simulink model "TST_InjVlv_BlkSht"  (R2016b)
settings: Solver=FixedStepDiscrete  StartTime=0.0  StopTime=simTime  FixedStep=sampleTime  RelTol=1e-3
values from neighbouring files (symbols this model uses):
  testCase = 1    [initTST_InjVlv_BlkSht_001.m]    (also in initTST_InjVlv_BlkSht_002.m = 2)
libraries: simulink x11, UnitTest_Lib x8
settings Model: Creator=zhengjinyan  LastModifiedBy=zhengjinyan
settings DebuggingCC: SignalRangeChecking=error

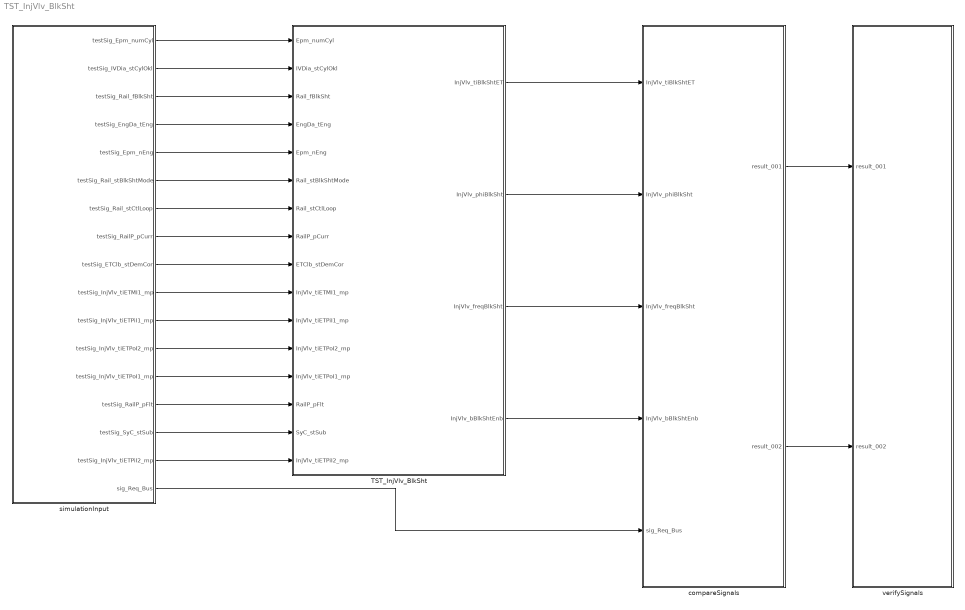
== system TST_InjVlv_BlkSht ==
  TST_InjVlv_BlkSht : Subsystem
  compareSignals : Subsystem
  simulationInput : Subsystem
  verifySignals : Subsystem
  wires:
  simulationInput/1(testSig_Epm_numCyl) -> TST_InjVlv_BlkSht/1(Epm_numCyl)
  simulationInput/2(testSig_IVDia_stCylOkl) -> TST_InjVlv_BlkSht/2(IVDia_stCylOkl)
  simulationInput/3(testSig_Rail_fBlkSht) -> TST_InjVlv_BlkSht/3(Rail_fBlkSht)
  simulationInput/4(testSig_EngDa_tEng) -> TST_InjVlv_BlkSht/4(EngDa_tEng)
  simulationInput/5(testSig_Epm_nEng) -> TST_InjVlv_BlkSht/5(Epm_nEng)
  simulationInput/6(testSig_Rail_stBlkShtMode) -> TST_InjVlv_BlkSht/6(Rail_stBlkShtMode)
  simulationInput/7(testSig_Rail_stCtlLoop) -> TST_InjVlv_BlkSht/7(Rail_stCtlLoop)
  simulationInput/8(testSig_RailP_pCurr) -> TST_InjVlv_BlkSht/8(RailP_pCurr)
  simulationInput/9(testSig_ETClb_stDemCor) -> TST_InjVlv_BlkSht/9(ETClb_stDemCor)
  simulationInput/10(testSig_InjVlv_tiETMI1_mp) -> TST_InjVlv_BlkSht/10(InjVlv_tiETMI1_mp)
  simulationInput/11(testSig_InjVlv_tiETPiI1_mp) -> TST_InjVlv_BlkSht/11(InjVlv_tiETPiI1_mp)
  simulationInput/12(testSig_InjVlv_tiETPoI2_mp) -> TST_InjVlv_BlkSht/12(InjVlv_tiETPoI2_mp)
  simulationInput/13(testSig_InjVlv_tiETPoI1_mp) -> TST_InjVlv_BlkSht/13(InjVlv_tiETPoI1_mp)
  simulationInput/14(testSig_RailP_pFlt) -> TST_InjVlv_BlkSht/14(RailP_pFlt)
  simulationInput/15(testSig_SyC_stSub) -> TST_InjVlv_BlkSht/15(SyC_stSub)
  simulationInput/16(testSig_InjVlv_tiETPiI2_mp) -> TST_InjVlv_BlkSht/16(InjVlv_tiETPiI2_mp)
  TST_InjVlv_BlkSht/1(InjVlv_tiBlkShtET) -> compareSignals/1(InjVlv_tiBlkShtET)
  TST_InjVlv_BlkSht/2(InjVlv_phiBlkSht) -> compareSignals/2(InjVlv_phiBlkSht)
  TST_InjVlv_BlkSht/3(InjVlv_freqBlkSht) -> compareSignals/3(InjVlv_freqBlkSht)
  TST_InjVlv_BlkSht/4(InjVlv_bBlkShtEnb) -> compareSignals/4(InjVlv_bBlkShtEnb)
  simulationInput/17(sig_Req_Bus) -> compareSignals/5(sig_Req_Bus)
  compareSignals/1(result_001) -> verifySignals/1(result_001)
  compareSignals/2(result_002) -> verifySignals/2(result_002)

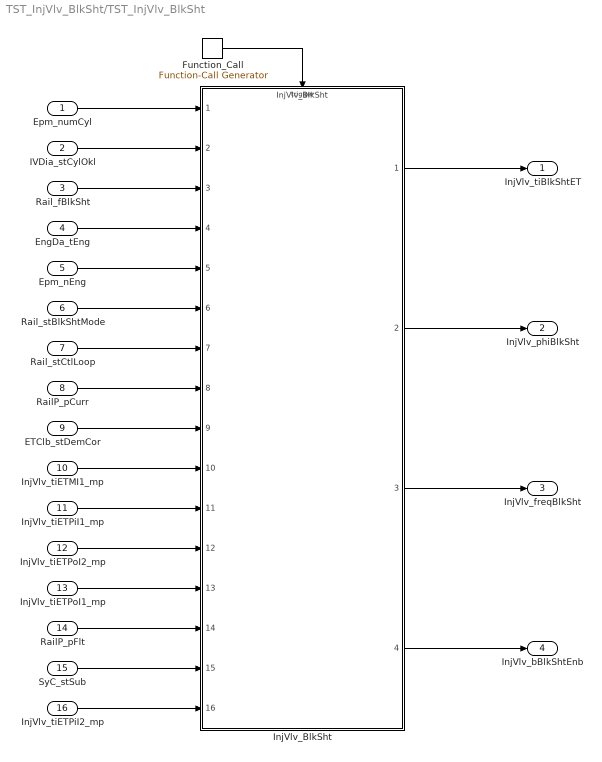
== system TST_InjVlv_BlkSht/TST_InjVlv_BlkSht ==
  Epm_numCyl : Inport
  IVDia_stCylOkl : Inport  Port=2
  Rail_fBlkSht : Inport  Port=3
  EngDa_tEng : Inport  Port=4
  Epm_nEng : Inport  Port=5
  Rail_stBlkShtMode : Inport  Port=6
  Rail_stCtlLoop : Inport  Port=7
  RailP_pCurr : Inport  Port=8
  ETClb_stDemCor : Inport  Port=9
  InjVlv_tiETMI1_mp : Inport  Port=10
  InjVlv_tiETPiI1_mp : Inport  Port=11
  InjVlv_tiETPoI2_mp : Inport  Port=12
  InjVlv_tiETPoI1_mp : Inport  Port=13
  RailP_pFlt : Inport  Port=14
  SyC_stSub : Inport  Port=15
  InjVlv_tiETPiI2_mp : Inport  Port=16
  Function_Call : simulink/Ports & Subsystems/Function-Call Generator  sample_time=sampleTime  numberOfIterations=1
  InjVlv_BlkSht : ModelReference  ModelNameDialog=InjVlv_BlkSht  SimulationMode=Normal  ModelReferenceVersion=1.63  TriggerPortName=function  TriggerPortTriggerType=function-call  TriggerPortStatesWhenEnabling=held
  InjVlv_tiBlkShtET : Outport
  InjVlv_phiBlkSht : Outport  Port=2
  InjVlv_freqBlkSht : Outport  Port=3
  InjVlv_bBlkShtEnb : Outport  Port=4
  wires:
  Function_Call/1 -> InjVlv_BlkSht/Trigger
  Epm_numCyl/1 -> InjVlv_BlkSht/1
  IVDia_stCylOkl/1 -> InjVlv_BlkSht/2
  Rail_fBlkSht/1 -> InjVlv_BlkSht/3
  EngDa_tEng/1 -> InjVlv_BlkSht/4
  Epm_nEng/1 -> InjVlv_BlkSht/5
  Rail_stBlkShtMode/1 -> InjVlv_BlkSht/6
  Rail_stCtlLoop/1 -> InjVlv_BlkSht/7
  RailP_pCurr/1 -> InjVlv_BlkSht/8
  ETClb_stDemCor/1 -> InjVlv_BlkSht/9
  InjVlv_tiETMI1_mp/1 -> InjVlv_BlkSht/10
  InjVlv_tiETPiI1_mp/1 -> InjVlv_BlkSht/11
  InjVlv_tiETPoI2_mp/1 -> InjVlv_BlkSht/12
  InjVlv_tiETPoI1_mp/1 -> InjVlv_BlkSht/13
  RailP_pFlt/1 -> InjVlv_BlkSht/14
  SyC_stSub/1 -> InjVlv_BlkSht/15
  InjVlv_tiETPiI2_mp/1 -> InjVlv_BlkSht/16
  InjVlv_BlkSht/1 -> InjVlv_tiBlkShtET/1
  InjVlv_BlkSht/2 -> InjVlv_phiBlkSht/1
  InjVlv_BlkSht/3 -> InjVlv_freqBlkSht/1
  InjVlv_BlkSht/4 -> InjVlv_bBlkShtEnb/1

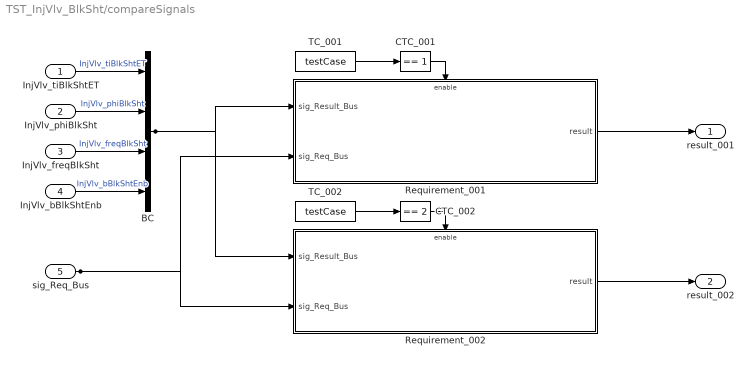
== system TST_InjVlv_BlkSht/compareSignals ==
  InjVlv_tiBlkShtET : Inport
  InjVlv_phiBlkSht : Inport  Port=2
  InjVlv_freqBlkSht : Inport  Port=3
  InjVlv_bBlkShtEnb : Inport  Port=4
  sig_Req_Bus : Inport  Port=5
  BC : BusCreator  Inputs=4
  CTC_001 : simulink/Logic and Bit Operations/Compare To Constant  relop===  const=1  OutDataTypeStr=boolean
  CTC_002 : simulink/Logic and Bit Operations/Compare To Constant  relop===  const=2  OutDataTypeStr=boolean
  Requirement_001 : Subsystem
  Requirement_002 : Subsystem
  TC_001 : Constant  Value=testCase
  TC_002 : Constant  Value=testCase
  result_001 : Outport
  result_002 : Outport  Port=2
  wires:
  InjVlv_tiBlkShtET/1 -> BC/1  "InjVlv_tiBlkShtET"
  InjVlv_phiBlkSht/1 -> BC/2  "InjVlv_phiBlkSht"
  InjVlv_freqBlkSht/1 -> BC/3  "InjVlv_freqBlkSht"
  InjVlv_bBlkShtEnb/1 -> BC/4  "InjVlv_bBlkShtEnb"
  TC_001/1 -> CTC_001/1
  CTC_001/1 -> Requirement_001/Enable
  sig_Req_Bus/1 -> Requirement_001/2(sig_Req_Bus), Requirement_002/2(sig_Req_Bus)
  BC/1 -> Requirement_001/1(sig_Result_Bus), Requirement_002/1(sig_Result_Bus)
  Requirement_001/1(result) -> result_001/1
  TC_002/1 -> CTC_002/1
  CTC_002/1 -> Requirement_002/Enable
  Requirement_002/1(result) -> result_002/1

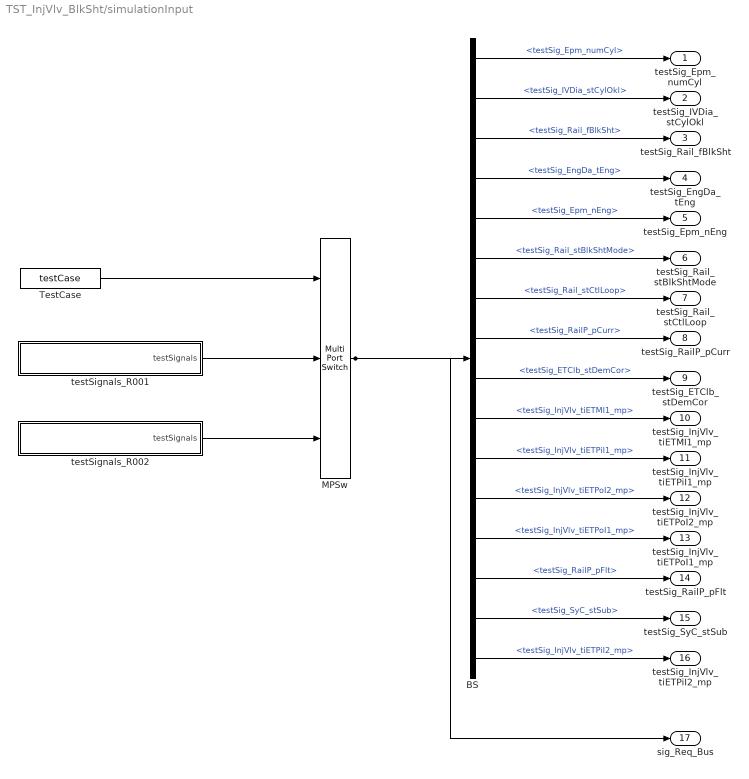
== system TST_InjVlv_BlkSht/simulationInput ==
  BS : BusSelector  OutputSignals=testSig_Epm_numCyl,testSig_IVDia_stCylOkl,testSig_Rail_fBlkSht,testSig_EngDa_tEng,testSig_Epm_nEng,testSig_Rail_stBlkShtMode,testSig_Rail_stCtlLoop,testSig_RailP_pCurr,testSig_ETClb_stDemCor,testSig_InjVlv_tiETMI1_mp,testSig_InjVlv_tiETPiI1_mp,testSig_InjVlv_tiETPoI2_mp,testSig_InjVlv_tiETPoI1_mp,testSig_RailP_pFlt,testSig_SyC_stSub,testSig_InjVlv_tiETPiI2_mp
  MPSw : MultiPortSwitch  Inputs=2  SaturateOnIntegerOverflow=on  InputSameDT=on
  TestCase : Constant  Value=testCase
  testSignals_R001 : Subsystem
  testSignals_R002 : Subsystem
  testSig_Epm_numCyl : Outport
  testSig_IVDia_stCylOkl : Outport  Port=2
  testSig_Rail_fBlkSht : Outport  Port=3
  testSig_EngDa_tEng : Outport  Port=4
  testSig_Epm_nEng : Outport  Port=5
  testSig_Rail_stBlkShtMode : Outport  Port=6
  testSig_Rail_stCtlLoop : Outport  Port=7
  testSig_RailP_pCurr : Outport  Port=8
  testSig_ETClb_stDemCor : Outport  Port=9
  testSig_InjVlv_tiETMI1_mp : Outport  Port=10
  testSig_InjVlv_tiETPiI1_mp : Outport  Port=11
  testSig_InjVlv_tiETPoI2_mp : Outport  Port=12
  testSig_InjVlv_tiETPoI1_mp : Outport  Port=13
  testSig_RailP_pFlt : Outport  Port=14
  testSig_SyC_stSub : Outport  Port=15
  testSig_InjVlv_tiETPiI2_mp : Outport  Port=16
  sig_Req_Bus : Outport  Port=17
  wires:
  BS/1 -> testSig_Epm_numCyl/1  "<testSig_Epm_numCyl>"
  BS/2 -> testSig_IVDia_stCylOkl/1  "<testSig_IVDia_stCylOkl>"
  BS/3 -> testSig_Rail_fBlkSht/1  "<testSig_Rail_fBlkSht>"
  BS/4 -> testSig_EngDa_tEng/1  "<testSig_EngDa_tEng>"
  BS/5 -> testSig_Epm_nEng/1  "<testSig_Epm_nEng>"
  BS/6 -> testSig_Rail_stBlkShtMode/1  "<testSig_Rail_stBlkShtMode>"
  BS/7 -> testSig_Rail_stCtlLoop/1  "<testSig_Rail_stCtlLoop>"
  BS/8 -> testSig_RailP_pCurr/1  "<testSig_RailP_pCurr>"
  BS/9 -> testSig_ETClb_stDemCor/1  "<testSig_ETClb_stDemCor>"
  BS/10 -> testSig_InjVlv_tiETMI1_mp/1  "<testSig_InjVlv_tiETMI1_mp>"
  BS/11 -> testSig_InjVlv_tiETPiI1_mp/1  "<testSig_InjVlv_tiETPiI1_mp>"
  BS/12 -> testSig_InjVlv_tiETPoI2_mp/1  "<testSig_InjVlv_tiETPoI2_mp>"
  BS/13 -> testSig_InjVlv_tiETPoI1_mp/1  "<testSig_InjVlv_tiETPoI1_mp>"
  BS/14 -> testSig_RailP_pFlt/1  "<testSig_RailP_pFlt>"
  BS/15 -> testSig_SyC_stSub/1  "<testSig_SyC_stSub>"
  BS/16 -> testSig_InjVlv_tiETPiI2_mp/1  "<testSig_InjVlv_tiETPiI2_mp>"
  MPSw/1 -> BS/1, sig_Req_Bus/1
  TestCase/1 -> MPSw/1
  testSignals_R001/1(testSignals) -> MPSw/2
  testSignals_R002/1(testSignals) -> MPSw/3

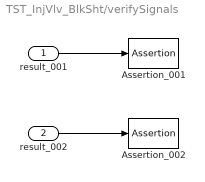
== system TST_InjVlv_BlkSht/verifySignals ==
  result_001 : Inport
  result_002 : Inport  Port=2
  Assertion_001 : Assertion  Enabled=off
  Assertion_002 : Assertion  Enabled=off
  wires:
  result_001/1 -> Assertion_001/1
  result_002/1 -> Assertion_002/1

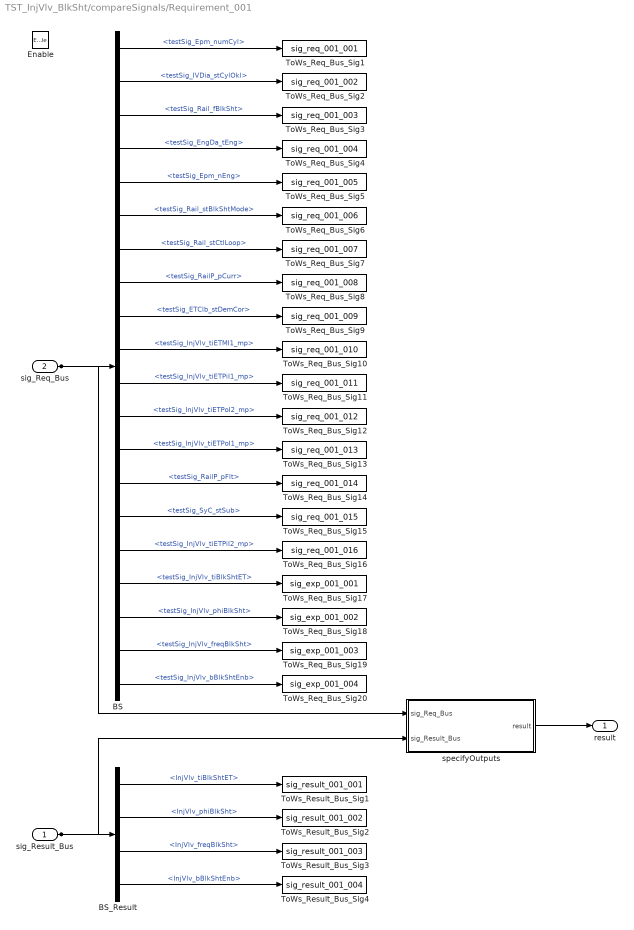
== system TST_InjVlv_BlkSht/compareSignals/Requirement_001 ==
  sig_Result_Bus : Inport
  sig_Req_Bus : Inport  Port=2
  Enable : EnablePort
  BS : BusSelector  OutputSignals=testSig_Epm_numCyl,testSig_IVDia_stCylOkl,testSig_Rail_fBlkSht,testSig_EngDa_tEng,testSig_Epm_nEng,testSig_Rail_stBlkShtMode,testSig_Rail_stCtlLoop,testSig_RailP_pCurr,testSig_ETClb_stDemCor,testSig_InjVlv_tiETMI1_mp,testSig_InjVlv_tiETPiI1_mp,testSig_InjVlv_tiETPoI2_mp,testSig_InjVlv_tiETPoI1_mp,testSig_RailP_pFlt,testSig_SyC_stSub,testSig_InjVlv_tiETPiI2_mp,testSig_InjVlv_tiBlkShtET,testSig_InjVlv_phiBlkSht,testSig_InjVlv_freqBlkSht,testSig_InjVlv_bBlkShtEnb
  BS_Result : BusSelector  OutputSignals=InjVlv_tiBlkShtET,InjVlv_phiBlkSht,InjVlv_freqBlkSht,InjVlv_bBlkShtEnb
  ToWs_Req_Bus_Sig1 : ToWorkspace  VariableName=sig_req_001_001  SaveFormat=Structure With Time
  ToWs_Req_Bus_Sig10 : ToWorkspace  VariableName=sig_req_001_010  SaveFormat=Structure With Time
  ToWs_Req_Bus_Sig11 : ToWorkspace  VariableName=sig_req_001_011  SaveFormat=Structure With Time
  ToWs_Req_Bus_Sig12 : ToWorkspace  VariableName=sig_req_001_012  SaveFormat=Structure With Time
  ToWs_Req_Bus_Sig13 : ToWorkspace  VariableName=sig_req_001_013  SaveFormat=Structure With Time
  ToWs_Req_Bus_Sig14 : ToWorkspace  VariableName=sig_req_001_014  SaveFormat=Structure With Time
  ToWs_Req_Bus_Sig15 : ToWorkspace  VariableName=sig_req_001_015  SaveFormat=Structure With Time
  ToWs_Req_Bus_Sig16 : ToWorkspace  VariableName=sig_req_001_016  SaveFormat=Structure With Time
  ToWs_Req_Bus_Sig17 : ToWorkspace  VariableName=sig_exp_001_001  SaveFormat=Structure With Time
  ToWs_Req_Bus_Sig18 : ToWorkspace  VariableName=sig_exp_001_002  SaveFormat=Structure With Time
  ToWs_Req_Bus_Sig19 : ToWorkspace  VariableName=sig_exp_001_003  SaveFormat=Structure With Time
  ToWs_Req_Bus_Sig2 : ToWorkspace  VariableName=sig_req_001_002  SaveFormat=Structure With Time
  ToWs_Req_Bus_Sig20 : ToWorkspace  VariableName=sig_exp_001_004  SaveFormat=Structure With Time
  ToWs_Req_Bus_Sig3 : ToWorkspace  VariableName=sig_req_001_003  SaveFormat=Structure With Time
  ToWs_Req_Bus_Sig4 : ToWorkspace  VariableName=sig_req_001_004  SaveFormat=Structure With Time
  ToWs_Req_Bus_Sig5 : ToWorkspace  VariableName=sig_req_001_005  SaveFormat=Structure With Time
  ToWs_Req_Bus_Sig6 : ToWorkspace  VariableName=sig_req_001_006  SaveFormat=Structure With Time
  ToWs_Req_Bus_Sig7 : ToWorkspace  VariableName=sig_req_001_007  SaveFormat=Structure With Time
  ToWs_Req_Bus_Sig8 : ToWorkspace  VariableName=sig_req_001_008  SaveFormat=Structure With Time
  ToWs_Req_Bus_Sig9 : ToWorkspace  VariableName=sig_req_001_009  SaveFormat=Structure With Time
  ToWs_Result_Bus_Sig1 : ToWorkspace  VariableName=sig_result_001_001  SaveFormat=Structure With Time
  ToWs_Result_Bus_Sig2 : ToWorkspace  VariableName=sig_result_001_002  SaveFormat=Structure With Time
  ToWs_Result_Bus_Sig3 : ToWorkspace  VariableName=sig_result_001_003  SaveFormat=Structure With Time
  ToWs_Result_Bus_Sig4 : ToWorkspace  VariableName=sig_result_001_004  SaveFormat=Structure With Time
  specifyOutputs : Subsystem
  result : Outport
  wires:
  sig_Req_Bus/1 -> BS/1, specifyOutputs/1(sig_Req_Bus)
  BS/1 -> ToWs_Req_Bus_Sig1/1  "<testSig_Epm_numCyl>"
  BS/2 -> ToWs_Req_Bus_Sig2/1  "<testSig_IVDia_stCylOkl>"
  BS/3 -> ToWs_Req_Bus_Sig3/1  "<testSig_Rail_fBlkSht>"
  BS/4 -> ToWs_Req_Bus_Sig4/1  "<testSig_EngDa_tEng>"
  BS/5 -> ToWs_Req_Bus_Sig5/1  "<testSig_Epm_nEng>"
  BS/6 -> ToWs_Req_Bus_Sig6/1  "<testSig_Rail_stBlkShtMode>"
  BS/7 -> ToWs_Req_Bus_Sig7/1  "<testSig_Rail_stCtlLoop>"
  BS/8 -> ToWs_Req_Bus_Sig8/1  "<testSig_RailP_pCurr>"
  BS/9 -> ToWs_Req_Bus_Sig9/1  "<testSig_ETClb_stDemCor>"
  BS/10 -> ToWs_Req_Bus_Sig10/1  "<testSig_InjVlv_tiETMI1_mp>"
  BS/11 -> ToWs_Req_Bus_Sig11/1  "<testSig_InjVlv_tiETPiI1_mp>"
  BS/12 -> ToWs_Req_Bus_Sig12/1  "<testSig_InjVlv_tiETPoI2_mp>"
  BS/13 -> ToWs_Req_Bus_Sig13/1  "<testSig_InjVlv_tiETPoI1_mp>"
  BS/14 -> ToWs_Req_Bus_Sig14/1  "<testSig_RailP_pFlt>"
  BS/15 -> ToWs_Req_Bus_Sig15/1  "<testSig_SyC_stSub>"
  BS/16 -> ToWs_Req_Bus_Sig16/1  "<testSig_InjVlv_tiETPiI2_mp>"
  BS/17 -> ToWs_Req_Bus_Sig17/1  "<testSig_InjVlv_tiBlkShtET>"
  BS/18 -> ToWs_Req_Bus_Sig18/1  "<testSig_InjVlv_phiBlkSht>"
  BS/19 -> ToWs_Req_Bus_Sig19/1  "<testSig_InjVlv_freqBlkSht>"
  BS/20 -> ToWs_Req_Bus_Sig20/1  "<testSig_InjVlv_bBlkShtEnb>"
  sig_Result_Bus/1 -> BS_Result/1, specifyOutputs/2(sig_Result_Bus)
  BS_Result/1 -> ToWs_Result_Bus_Sig1/1  "<InjVlv_tiBlkShtET>"
  BS_Result/2 -> ToWs_Result_Bus_Sig2/1  "<InjVlv_phiBlkSht>"
  BS_Result/3 -> ToWs_Result_Bus_Sig3/1  "<InjVlv_freqBlkSht>"
  BS_Result/4 -> ToWs_Result_Bus_Sig4/1  "<InjVlv_bBlkShtEnb>"
  specifyOutputs/1(result) -> result/1

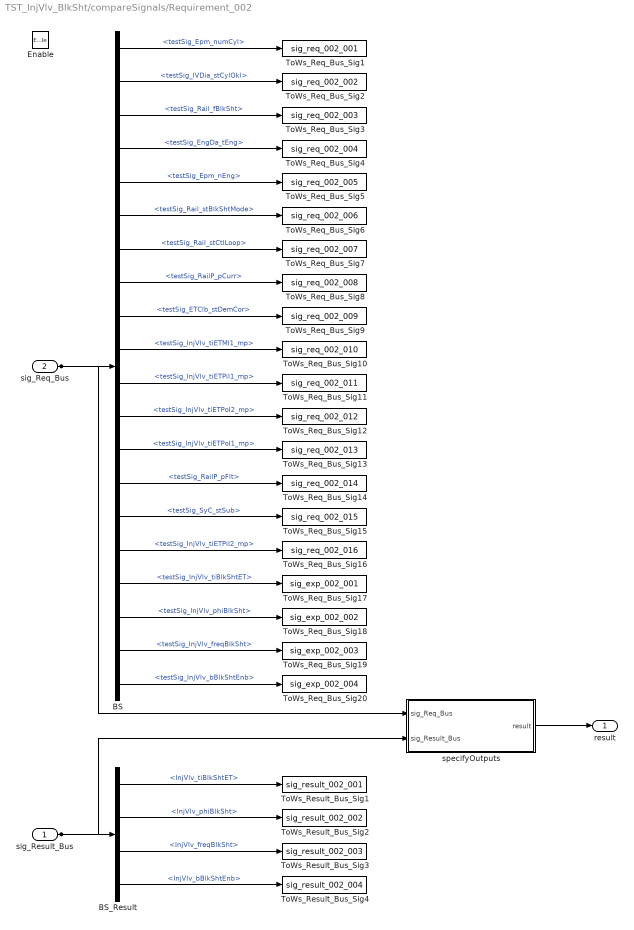
== system TST_InjVlv_BlkSht/compareSignals/Requirement_002 ==
  sig_Result_Bus : Inport
  sig_Req_Bus : Inport  Port=2
  Enable : EnablePort
  BS : BusSelector  OutputSignals=testSig_Epm_numCyl,testSig_IVDia_stCylOkl,testSig_Rail_fBlkSht,testSig_EngDa_tEng,testSig_Epm_nEng,testSig_Rail_stBlkShtMode,testSig_Rail_stCtlLoop,testSig_RailP_pCurr,testSig_ETClb_stDemCor,testSig_InjVlv_tiETMI1_mp,testSig_InjVlv_tiETPiI1_mp,testSig_InjVlv_tiETPoI2_mp,testSig_InjVlv_tiETPoI1_mp,testSig_RailP_pFlt,testSig_SyC_stSub,testSig_InjVlv_tiETPiI2_mp,testSig_InjVlv_tiBlkShtET,testSig_InjVlv_phiBlkSht,testSig_InjVlv_freqBlkSht,testSig_InjVlv_bBlkShtEnb
  BS_Result : BusSelector  OutputSignals=InjVlv_tiBlkShtET,InjVlv_phiBlkSht,InjVlv_freqBlkSht,InjVlv_bBlkShtEnb
  ToWs_Req_Bus_Sig1 : ToWorkspace  VariableName=sig_req_002_001  SaveFormat=Structure With Time
  ToWs_Req_Bus_Sig10 : ToWorkspace  VariableName=sig_req_002_010  SaveFormat=Structure With Time
  ToWs_Req_Bus_Sig11 : ToWorkspace  VariableName=sig_req_002_011  SaveFormat=Structure With Time
  ToWs_Req_Bus_Sig12 : ToWorkspace  VariableName=sig_req_002_012  SaveFormat=Structure With Time
  ToWs_Req_Bus_Sig13 : ToWorkspace  VariableName=sig_req_002_013  SaveFormat=Structure With Time
  ToWs_Req_Bus_Sig14 : ToWorkspace  VariableName=sig_req_002_014  SaveFormat=Structure With Time
  ToWs_Req_Bus_Sig15 : ToWorkspace  VariableName=sig_req_002_015  SaveFormat=Structure With Time
  ToWs_Req_Bus_Sig16 : ToWorkspace  VariableName=sig_req_002_016  SaveFormat=Structure With Time
  ToWs_Req_Bus_Sig17 : ToWorkspace  VariableName=sig_exp_002_001  SaveFormat=Structure With Time
  ToWs_Req_Bus_Sig18 : ToWorkspace  VariableName=sig_exp_002_002  SaveFormat=Structure With Time
  ToWs_Req_Bus_Sig19 : ToWorkspace  VariableName=sig_exp_002_003  SaveFormat=Structure With Time
  ToWs_Req_Bus_Sig2 : ToWorkspace  VariableName=sig_req_002_002  SaveFormat=Structure With Time
  ToWs_Req_Bus_Sig20 : ToWorkspace  VariableName=sig_exp_002_004  SaveFormat=Structure With Time
  ToWs_Req_Bus_Sig3 : ToWorkspace  VariableName=sig_req_002_003  SaveFormat=Structure With Time
  ToWs_Req_Bus_Sig4 : ToWorkspace  VariableName=sig_req_002_004  SaveFormat=Structure With Time
  ToWs_Req_Bus_Sig5 : ToWorkspace  VariableName=sig_req_002_005  SaveFormat=Structure With Time
  ToWs_Req_Bus_Sig6 : ToWorkspace  VariableName=sig_req_002_006  SaveFormat=Structure With Time
  ToWs_Req_Bus_Sig7 : ToWorkspace  VariableName=sig_req_002_007  SaveFormat=Structure With Time
  ToWs_Req_Bus_Sig8 : ToWorkspace  VariableName=sig_req_002_008  SaveFormat=Structure With Time
  ToWs_Req_Bus_Sig9 : ToWorkspace  VariableName=sig_req_002_009  SaveFormat=Structure With Time
  ToWs_Result_Bus_Sig1 : ToWorkspace  VariableName=sig_result_002_001  SaveFormat=Structure With Time
  ToWs_Result_Bus_Sig2 : ToWorkspace  VariableName=sig_result_002_002  SaveFormat=Structure With Time
  ToWs_Result_Bus_Sig3 : ToWorkspace  VariableName=sig_result_002_003  SaveFormat=Structure With Time
  ToWs_Result_Bus_Sig4 : ToWorkspace  VariableName=sig_result_002_004  SaveFormat=Structure With Time
  specifyOutputs : Subsystem
  result : Outport
  wires:
  sig_Req_Bus/1 -> BS/1, specifyOutputs/1(sig_Req_Bus)
  BS/1 -> ToWs_Req_Bus_Sig1/1  "<testSig_Epm_numCyl>"
  BS/2 -> ToWs_Req_Bus_Sig2/1  "<testSig_IVDia_stCylOkl>"
  BS/3 -> ToWs_Req_Bus_Sig3/1  "<testSig_Rail_fBlkSht>"
  BS/4 -> ToWs_Req_Bus_Sig4/1  "<testSig_EngDa_tEng>"
  BS/5 -> ToWs_Req_Bus_Sig5/1  "<testSig_Epm_nEng>"
  BS/6 -> ToWs_Req_Bus_Sig6/1  "<testSig_Rail_stBlkShtMode>"
  BS/7 -> ToWs_Req_Bus_Sig7/1  "<testSig_Rail_stCtlLoop>"
  BS/8 -> ToWs_Req_Bus_Sig8/1  "<testSig_RailP_pCurr>"
  BS/9 -> ToWs_Req_Bus_Sig9/1  "<testSig_ETClb_stDemCor>"
  BS/10 -> ToWs_Req_Bus_Sig10/1  "<testSig_InjVlv_tiETMI1_mp>"
  BS/11 -> ToWs_Req_Bus_Sig11/1  "<testSig_InjVlv_tiETPiI1_mp>"
  BS/12 -> ToWs_Req_Bus_Sig12/1  "<testSig_InjVlv_tiETPoI2_mp>"
  BS/13 -> ToWs_Req_Bus_Sig13/1  "<testSig_InjVlv_tiETPoI1_mp>"
  BS/14 -> ToWs_Req_Bus_Sig14/1  "<testSig_RailP_pFlt>"
  BS/15 -> ToWs_Req_Bus_Sig15/1  "<testSig_SyC_stSub>"
  BS/16 -> ToWs_Req_Bus_Sig16/1  "<testSig_InjVlv_tiETPiI2_mp>"
  BS/17 -> ToWs_Req_Bus_Sig17/1  "<testSig_InjVlv_tiBlkShtET>"
  BS/18 -> ToWs_Req_Bus_Sig18/1  "<testSig_InjVlv_phiBlkSht>"
  BS/19 -> ToWs_Req_Bus_Sig19/1  "<testSig_InjVlv_freqBlkSht>"
  BS/20 -> ToWs_Req_Bus_Sig20/1  "<testSig_InjVlv_bBlkShtEnb>"
  sig_Result_Bus/1 -> BS_Result/1, specifyOutputs/2(sig_Result_Bus)
  BS_Result/1 -> ToWs_Result_Bus_Sig1/1  "<InjVlv_tiBlkShtET>"
  BS_Result/2 -> ToWs_Result_Bus_Sig2/1  "<InjVlv_phiBlkSht>"
  BS_Result/3 -> ToWs_Result_Bus_Sig3/1  "<InjVlv_freqBlkSht>"
  BS_Result/4 -> ToWs_Result_Bus_Sig4/1  "<InjVlv_bBlkShtEnb>"
  specifyOutputs/1(result) -> result/1

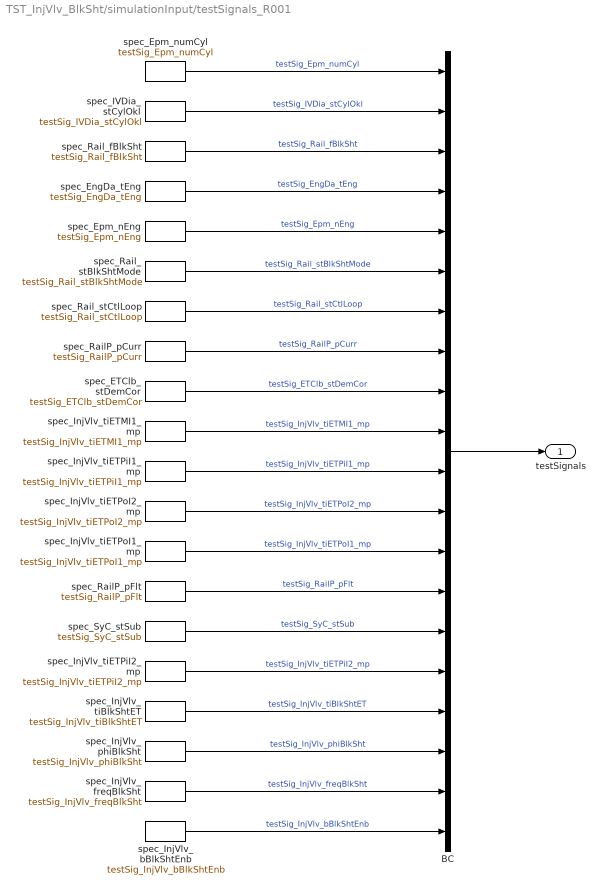
== system TST_InjVlv_BlkSht/simulationInput/testSignals_R001 ==
  BC : BusCreator  Inputs=20
  spec_ETClb_stDemCor : FromWorkspace  VariableName=testSig_ETClb_stDemCor  Interpolate=off  OutputAfterFinalValue=Holding final value
  spec_EngDa_tEng : FromWorkspace  VariableName=testSig_EngDa_tEng  Interpolate=off  OutputAfterFinalValue=Holding final value
  spec_Epm_nEng : FromWorkspace  VariableName=testSig_Epm_nEng  Interpolate=off  OutputAfterFinalValue=Holding final value
  spec_Epm_numCyl : FromWorkspace  VariableName=testSig_Epm_numCyl  Interpolate=off  OutputAfterFinalValue=Holding final value
  spec_IVDia_stCylOkl : FromWorkspace  VariableName=testSig_IVDia_stCylOkl  Interpolate=off  OutputAfterFinalValue=Holding final value
  spec_InjVlv_bBlkShtEnb : FromWorkspace  VariableName=testSig_InjVlv_bBlkShtEnb  Interpolate=off  OutputAfterFinalValue=Holding final value
  spec_InjVlv_freqBlkSht : FromWorkspace  VariableName=testSig_InjVlv_freqBlkSht  Interpolate=off  OutputAfterFinalValue=Holding final value
  spec_InjVlv_phiBlkSht : FromWorkspace  VariableName=testSig_InjVlv_phiBlkSht  Interpolate=off  OutputAfterFinalValue=Holding final value
  spec_InjVlv_tiBlkShtET : FromWorkspace  VariableName=testSig_InjVlv_tiBlkShtET  Interpolate=off  OutputAfterFinalValue=Holding final value
  spec_InjVlv_tiETMI1_mp : FromWorkspace  VariableName=testSig_InjVlv_tiETMI1_mp  Interpolate=off  OutputAfterFinalValue=Holding final value
  spec_InjVlv_tiETPiI1_mp : FromWorkspace  VariableName=testSig_InjVlv_tiETPiI1_mp  Interpolate=off  OutputAfterFinalValue=Holding final value
  spec_InjVlv_tiETPiI2_mp : FromWorkspace  VariableName=testSig_InjVlv_tiETPiI2_mp  Interpolate=off  OutputAfterFinalValue=Holding final value
  spec_InjVlv_tiETPoI1_mp : FromWorkspace  VariableName=testSig_InjVlv_tiETPoI1_mp  Interpolate=off  OutputAfterFinalValue=Holding final value
  spec_InjVlv_tiETPoI2_mp : FromWorkspace  VariableName=testSig_InjVlv_tiETPoI2_mp  Interpolate=off  OutputAfterFinalValue=Holding final value
  spec_RailP_pCurr : FromWorkspace  VariableName=testSig_RailP_pCurr  Interpolate=off  OutputAfterFinalValue=Holding final value
  spec_RailP_pFlt : FromWorkspace  VariableName=testSig_RailP_pFlt  Interpolate=off  OutputAfterFinalValue=Holding final value
  spec_Rail_fBlkSht : FromWorkspace  VariableName=testSig_Rail_fBlkSht  Interpolate=off  OutputAfterFinalValue=Holding final value
  spec_Rail_stBlkShtMode : FromWorkspace  VariableName=testSig_Rail_stBlkShtMode  Interpolate=off  OutputAfterFinalValue=Holding final value
  spec_Rail_stCtlLoop : FromWorkspace  VariableName=testSig_Rail_stCtlLoop  Interpolate=off  OutputAfterFinalValue=Holding final value
  spec_SyC_stSub : FromWorkspace  VariableName=testSig_SyC_stSub  Interpolate=off  OutputAfterFinalValue=Holding final value
  testSignals : Outport
  wires:
  BC/1 -> testSignals/1
  spec_Epm_numCyl/1 -> BC/1  "testSig_Epm_numCyl"
  spec_IVDia_stCylOkl/1 -> BC/2  "testSig_IVDia_stCylOkl"
  spec_Rail_fBlkSht/1 -> BC/3  "testSig_Rail_fBlkSht"
  spec_EngDa_tEng/1 -> BC/4  "testSig_EngDa_tEng"
  spec_Epm_nEng/1 -> BC/5  "testSig_Epm_nEng"
  spec_Rail_stBlkShtMode/1 -> BC/6  "testSig_Rail_stBlkShtMode"
  spec_Rail_stCtlLoop/1 -> BC/7  "testSig_Rail_stCtlLoop"
  spec_RailP_pCurr/1 -> BC/8  "testSig_RailP_pCurr"
  spec_ETClb_stDemCor/1 -> BC/9  "testSig_ETClb_stDemCor"
  spec_InjVlv_tiETMI1_mp/1 -> BC/10  "testSig_InjVlv_tiETMI1_mp"
  spec_InjVlv_tiETPiI1_mp/1 -> BC/11  "testSig_InjVlv_tiETPiI1_mp"
  spec_InjVlv_tiETPoI2_mp/1 -> BC/12  "testSig_InjVlv_tiETPoI2_mp"
  spec_InjVlv_tiETPoI1_mp/1 -> BC/13  "testSig_InjVlv_tiETPoI1_mp"
  spec_RailP_pFlt/1 -> BC/14  "testSig_RailP_pFlt"
  spec_SyC_stSub/1 -> BC/15  "testSig_SyC_stSub"
  spec_InjVlv_tiETPiI2_mp/1 -> BC/16  "testSig_InjVlv_tiETPiI2_mp"
  spec_InjVlv_tiBlkShtET/1 -> BC/17  "testSig_InjVlv_tiBlkShtET"
  spec_InjVlv_phiBlkSht/1 -> BC/18  "testSig_InjVlv_phiBlkSht"
  spec_InjVlv_freqBlkSht/1 -> BC/19  "testSig_InjVlv_freqBlkSht"
  spec_InjVlv_bBlkShtEnb/1 -> BC/20  "testSig_InjVlv_bBlkShtEnb"

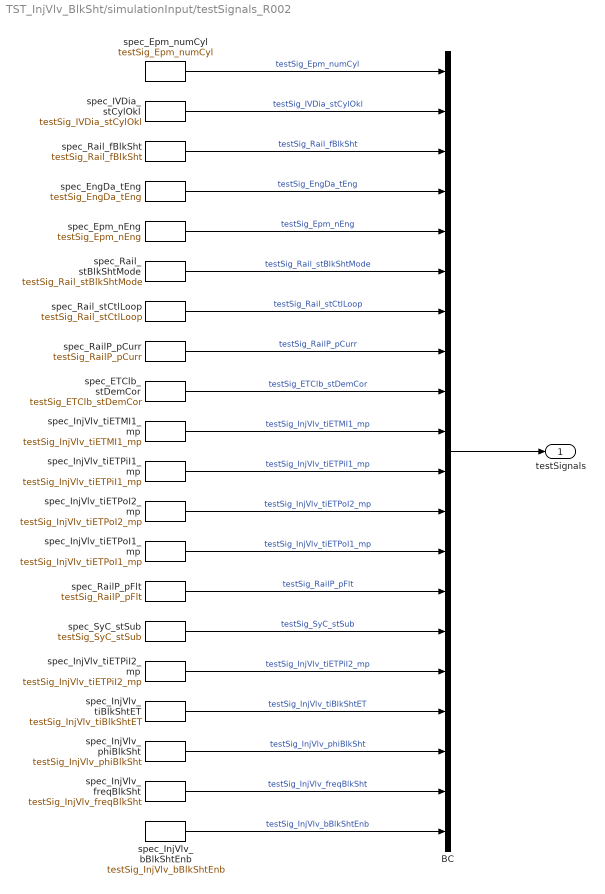
== system TST_InjVlv_BlkSht/simulationInput/testSignals_R002 ==
  BC : BusCreator  Inputs=20
  spec_ETClb_stDemCor : FromWorkspace  VariableName=testSig_ETClb_stDemCor  Interpolate=off  OutputAfterFinalValue=Holding final value
  spec_EngDa_tEng : FromWorkspace  VariableName=testSig_EngDa_tEng  Interpolate=off  OutputAfterFinalValue=Holding final value
  spec_Epm_nEng : FromWorkspace  VariableName=testSig_Epm_nEng  Interpolate=off  OutputAfterFinalValue=Holding final value
  spec_Epm_numCyl : FromWorkspace  VariableName=testSig_Epm_numCyl  Interpolate=off  OutputAfterFinalValue=Holding final value
  spec_IVDia_stCylOkl : FromWorkspace  VariableName=testSig_IVDia_stCylOkl  Interpolate=off  OutputAfterFinalValue=Holding final value
  spec_InjVlv_bBlkShtEnb : FromWorkspace  VariableName=testSig_InjVlv_bBlkShtEnb  Interpolate=off  OutputAfterFinalValue=Holding final value
  spec_InjVlv_freqBlkSht : FromWorkspace  VariableName=testSig_InjVlv_freqBlkSht  Interpolate=off  OutputAfterFinalValue=Holding final value
  spec_InjVlv_phiBlkSht : FromWorkspace  VariableName=testSig_InjVlv_phiBlkSht  Interpolate=off  OutputAfterFinalValue=Holding final value
  spec_InjVlv_tiBlkShtET : FromWorkspace  VariableName=testSig_InjVlv_tiBlkShtET  Interpolate=off  OutputAfterFinalValue=Holding final value
  spec_InjVlv_tiETMI1_mp : FromWorkspace  VariableName=testSig_InjVlv_tiETMI1_mp  Interpolate=off  OutputAfterFinalValue=Holding final value
  spec_InjVlv_tiETPiI1_mp : FromWorkspace  VariableName=testSig_InjVlv_tiETPiI1_mp  Interpolate=off  OutputAfterFinalValue=Holding final value
  spec_InjVlv_tiETPiI2_mp : FromWorkspace  VariableName=testSig_InjVlv_tiETPiI2_mp  Interpolate=off  OutputAfterFinalValue=Holding final value
  spec_InjVlv_tiETPoI1_mp : FromWorkspace  VariableName=testSig_InjVlv_tiETPoI1_mp  Interpolate=off  OutputAfterFinalValue=Holding final value
  spec_InjVlv_tiETPoI2_mp : FromWorkspace  VariableName=testSig_InjVlv_tiETPoI2_mp  Interpolate=off  OutputAfterFinalValue=Holding final value
  spec_RailP_pCurr : FromWorkspace  VariableName=testSig_RailP_pCurr  Interpolate=off  OutputAfterFinalValue=Holding final value
  spec_RailP_pFlt : FromWorkspace  VariableName=testSig_RailP_pFlt  Interpolate=off  OutputAfterFinalValue=Holding final value
  spec_Rail_fBlkSht : FromWorkspace  VariableName=testSig_Rail_fBlkSht  Interpolate=off  OutputAfterFinalValue=Holding final value
  spec_Rail_stBlkShtMode : FromWorkspace  VariableName=testSig_Rail_stBlkShtMode  Interpolate=off  OutputAfterFinalValue=Holding final value
  spec_Rail_stCtlLoop : FromWorkspace  VariableName=testSig_Rail_stCtlLoop  Interpolate=off  OutputAfterFinalValue=Holding final value
  spec_SyC_stSub : FromWorkspace  VariableName=testSig_SyC_stSub  Interpolate=off  OutputAfterFinalValue=Holding final value
  testSignals : Outport
  wires:
  BC/1 -> testSignals/1
  spec_Epm_numCyl/1 -> BC/1  "testSig_Epm_numCyl"
  spec_IVDia_stCylOkl/1 -> BC/2  "testSig_IVDia_stCylOkl"
  spec_Rail_fBlkSht/1 -> BC/3  "testSig_Rail_fBlkSht"
  spec_EngDa_tEng/1 -> BC/4  "testSig_EngDa_tEng"
  spec_Epm_nEng/1 -> BC/5  "testSig_Epm_nEng"
  spec_Rail_stBlkShtMode/1 -> BC/6  "testSig_Rail_stBlkShtMode"
  spec_Rail_stCtlLoop/1 -> BC/7  "testSig_Rail_stCtlLoop"
  spec_RailP_pCurr/1 -> BC/8  "testSig_RailP_pCurr"
  spec_ETClb_stDemCor/1 -> BC/9  "testSig_ETClb_stDemCor"
  spec_InjVlv_tiETMI1_mp/1 -> BC/10  "testSig_InjVlv_tiETMI1_mp"
  spec_InjVlv_tiETPiI1_mp/1 -> BC/11  "testSig_InjVlv_tiETPiI1_mp"
  spec_InjVlv_tiETPoI2_mp/1 -> BC/12  "testSig_InjVlv_tiETPoI2_mp"
  spec_InjVlv_tiETPoI1_mp/1 -> BC/13  "testSig_InjVlv_tiETPoI1_mp"
  spec_RailP_pFlt/1 -> BC/14  "testSig_RailP_pFlt"
  spec_SyC_stSub/1 -> BC/15  "testSig_SyC_stSub"
  spec_InjVlv_tiETPiI2_mp/1 -> BC/16  "testSig_InjVlv_tiETPiI2_mp"
  spec_InjVlv_tiBlkShtET/1 -> BC/17  "testSig_InjVlv_tiBlkShtET"
  spec_InjVlv_phiBlkSht/1 -> BC/18  "testSig_InjVlv_phiBlkSht"
  spec_InjVlv_freqBlkSht/1 -> BC/19  "testSig_InjVlv_freqBlkSht"
  spec_InjVlv_bBlkShtEnb/1 -> BC/20  "testSig_InjVlv_bBlkShtEnb"

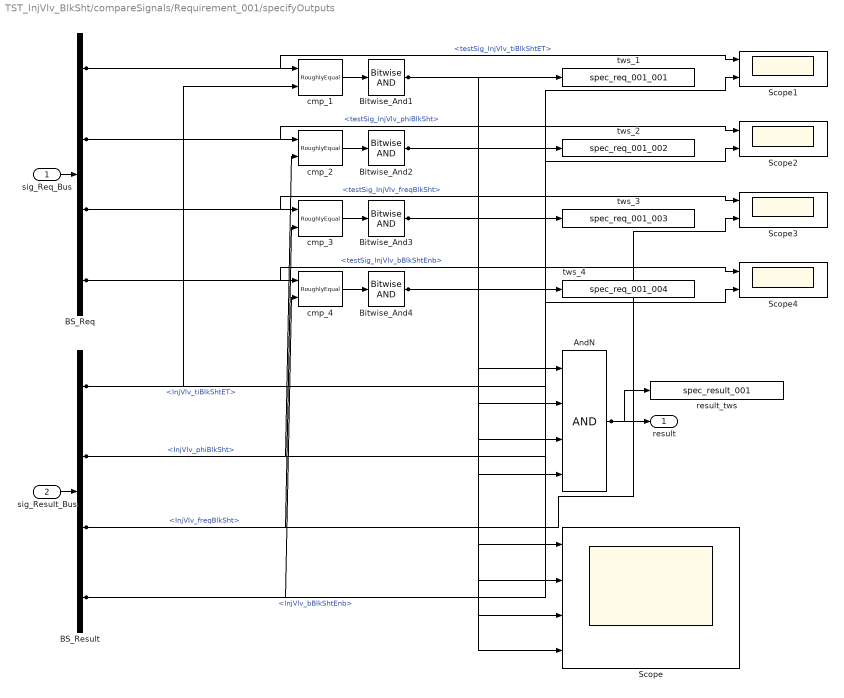
== system TST_InjVlv_BlkSht/compareSignals/Requirement_001/specifyOutputs ==
  sig_Req_Bus : Inport
  sig_Result_Bus : Inport  Port=2
  AndN : Logic  Inputs=4
  BS_Req : BusSelector  OutputSignals=testSig_InjVlv_tiBlkShtET,testSig_InjVlv_phiBlkSht,testSig_InjVlv_freqBlkSht,testSig_InjVlv_bBlkShtEnb
  BS_Result : BusSelector  OutputSignals=InjVlv_tiBlkShtET,InjVlv_phiBlkSht,InjVlv_freqBlkSht,InjVlv_bBlkShtEnb
  Bitwise_And{1..4} (4 alike) : simulink/Logic and Bit Operations/Bitwise Operator  logicop=AND  UseBitMask=off  BitMask=bin2dec('11011001')  BitMaskRealWorld=Stored Integer
  Scope : Scope  NumInputPorts=4
  Scope{1..4} (4 alike) : Scope  NumInputPorts=2
  cmp_{1..4} (4 alike) : UnitTest_Lib/RoughlyEqual  slope=0.1
  result_tws : ToWorkspace  VariableName=spec_result_001
  tws_1 : ToWorkspace  VariableName=spec_req_001_001
  tws_2 : ToWorkspace  VariableName=spec_req_001_002
  tws_3 : ToWorkspace  VariableName=spec_req_001_003
  tws_4 : ToWorkspace  VariableName=spec_req_001_004
  result : Outport
  wires:
  sig_Req_Bus/1 -> BS_Req/1
  sig_Result_Bus/1 -> BS_Result/1
  AndN/1 -> result/1, result_tws/1
  BS_Req/1 -> cmp_1/1, Scope1/1  "<testSig_InjVlv_tiBlkShtET>"
  BS_Result/1 -> cmp_1/2, Scope1/2  "<InjVlv_tiBlkShtET>"
  cmp_1/1 -> Bitwise_And1/1
  Bitwise_And1/1 -> tws_1/1, AndN/1, Scope/1
  BS_Req/2 -> cmp_2/1, Scope2/1  "<testSig_InjVlv_phiBlkSht>"
  BS_Result/2 -> cmp_2/2, Scope2/2  "<InjVlv_phiBlkSht>"
  cmp_2/1 -> Bitwise_And2/1
  Bitwise_And2/1 -> tws_2/1, AndN/2, Scope/2
  BS_Req/3 -> cmp_3/1, Scope3/1  "<testSig_InjVlv_freqBlkSht>"
  BS_Result/3 -> cmp_3/2, Scope3/2  "<InjVlv_freqBlkSht>"
  cmp_3/1 -> Bitwise_And3/1
  Bitwise_And3/1 -> tws_3/1, AndN/3, Scope/3
  BS_Req/4 -> cmp_4/1, Scope4/1  "<testSig_InjVlv_bBlkShtEnb>"
  BS_Result/4 -> cmp_4/2, Scope4/2  "<InjVlv_bBlkShtEnb>"
  cmp_4/1 -> Bitwise_And4/1
  Bitwise_And4/1 -> tws_4/1, AndN/4, Scope/4

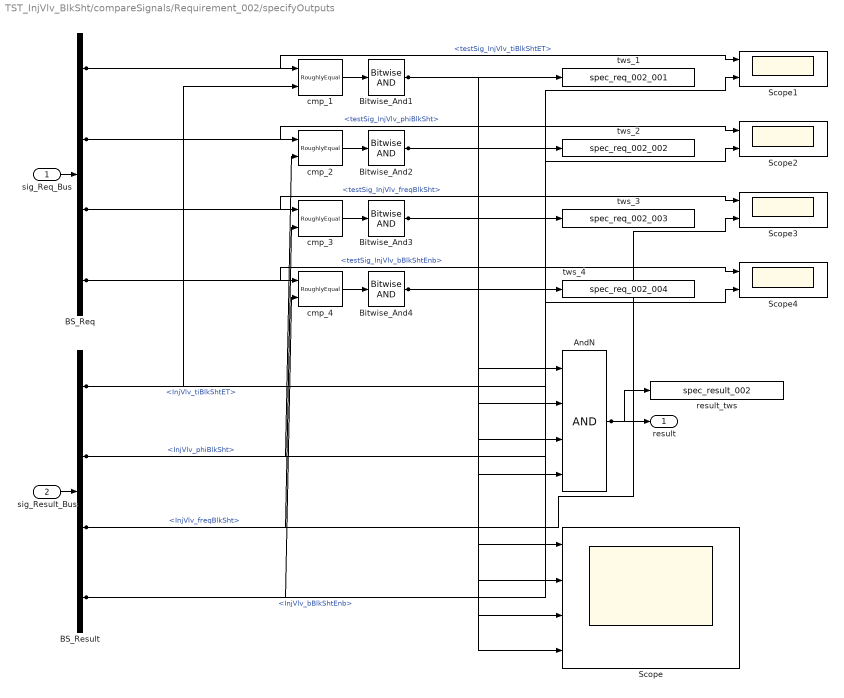
== system TST_InjVlv_BlkSht/compareSignals/Requirement_002/specifyOutputs ==
  sig_Req_Bus : Inport
  sig_Result_Bus : Inport  Port=2
  AndN : Logic  Inputs=4
  BS_Req : BusSelector  OutputSignals=testSig_InjVlv_tiBlkShtET,testSig_InjVlv_phiBlkSht,testSig_InjVlv_freqBlkSht,testSig_InjVlv_bBlkShtEnb
  BS_Result : BusSelector  OutputSignals=InjVlv_tiBlkShtET,InjVlv_phiBlkSht,InjVlv_freqBlkSht,InjVlv_bBlkShtEnb
  Bitwise_And{1..4} (4 alike) : simulink/Logic and Bit Operations/Bitwise Operator  logicop=AND  UseBitMask=off  BitMask=bin2dec('11011001')  BitMaskRealWorld=Stored Integer
  Scope : Scope  NumInputPorts=4
  Scope{1..4} (4 alike) : Scope  NumInputPorts=2
  cmp_{1..4} (4 alike) : UnitTest_Lib/RoughlyEqual  slope=0.1
  result_tws : ToWorkspace  VariableName=spec_result_002
  tws_1 : ToWorkspace  VariableName=spec_req_002_001
  tws_2 : ToWorkspace  VariableName=spec_req_002_002
  tws_3 : ToWorkspace  VariableName=spec_req_002_003
  tws_4 : ToWorkspace  VariableName=spec_req_002_004
  result : Outport
  wires:
  sig_Req_Bus/1 -> BS_Req/1
  sig_Result_Bus/1 -> BS_Result/1
  AndN/1 -> result/1, result_tws/1
  BS_Req/1 -> cmp_1/1, Scope1/1  "<testSig_InjVlv_tiBlkShtET>"
  BS_Result/1 -> cmp_1/2, Scope1/2  "<InjVlv_tiBlkShtET>"
  cmp_1/1 -> Bitwise_And1/1
  Bitwise_And1/1 -> tws_1/1, AndN/1, Scope/1
  BS_Req/2 -> cmp_2/1, Scope2/1  "<testSig_InjVlv_phiBlkSht>"
  BS_Result/2 -> cmp_2/2, Scope2/2  "<InjVlv_phiBlkSht>"
  cmp_2/1 -> Bitwise_And2/1
  Bitwise_And2/1 -> tws_2/1, AndN/2, Scope/2
  BS_Req/3 -> cmp_3/1, Scope3/1  "<testSig_InjVlv_freqBlkSht>"
  BS_Result/3 -> cmp_3/2, Scope3/2  "<InjVlv_freqBlkSht>"
  cmp_3/1 -> Bitwise_And3/1
  Bitwise_And3/1 -> tws_3/1, AndN/3, Scope/3
  BS_Req/4 -> cmp_4/1, Scope4/1  "<testSig_InjVlv_bBlkShtEnb>"
  BS_Result/4 -> cmp_4/2, Scope4/2  "<InjVlv_bBlkShtEnb>"
  cmp_4/1 -> Bitwise_And4/1
  Bitwise_And4/1 -> tws_4/1, AndN/4, Scope/4
